simulink model "hw1"  (R2022a)
settings: Solver=VariableStepAuto  StartTime=0.0  StopTime=40  RelTol=1e-3
settings Model: Creator=谢嵩  LastModifiedBy=谢嵩

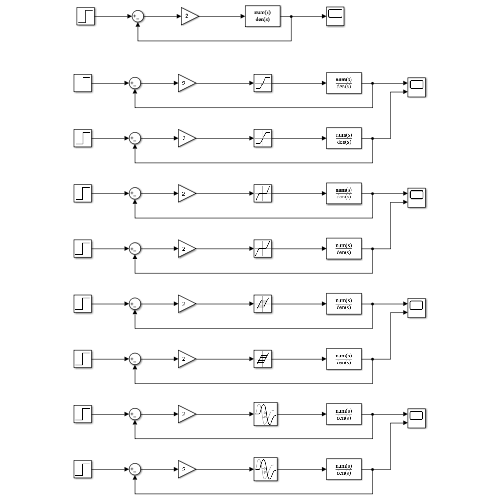
[thumbnail: Simulink's stored preview of the top-level diagram]
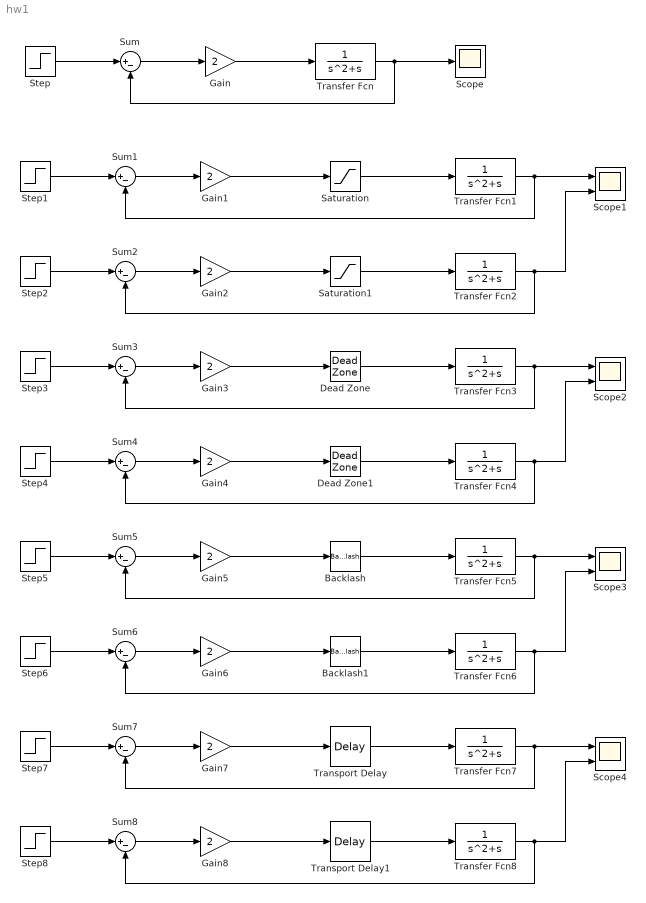
== system hw1 ==
  Backlash : Backlash
  Backlash1 : Backlash  BacklashWidth=0.4
  Dead Zone : DeadZone
  Dead Zone1 : DeadZone  LowerValue=-0.2  UpperValue=0.2
  Gain{,1..8} (9 alike) : Gain  Gain=2
  Saturation : Saturate
  Saturation1 : Saturate  UpperLimit=0.2  LowerLimit=-0.2
  Scope : Scope
  Scope{1..4} (4 alike) : Scope  NumInputPorts=2
  Step{,1..8} (9 alike) : Step  SampleTime=0
  Sum{,1..8} (9 alike) : Sum  Inputs=|+-
  Transfer Fcn{,1..8} (9 alike) : TransferFcn  Denominator=[1 1 0]
  Transport Delay : TransportDelay  DelayTime=0.5
  Transport Delay1 : TransportDelay  DelayTime=0.2
  wires:
  Step/1 -> Sum/1
  Sum/1 -> Gain/1
  Gain/1 -> Transfer Fcn/1
  Transfer Fcn/1 -> Sum/2, Scope/1
  Transfer Fcn1/1 -> Sum1/2, Scope1/1
  Step1/1 -> Sum1/1
  Sum1/1 -> Gain1/1
  Gain1/1 -> Saturation/1
  Saturation/1 -> Transfer Fcn1/1
  Transfer Fcn2/1 -> Scope1/2, Sum2/2
  Sum2/1 -> Gain2/1
  Saturation1/1 -> Transfer Fcn2/1
  Step2/1 -> Sum2/1
  Gain2/1 -> Saturation1/1
  Dead Zone/1 -> Transfer Fcn3/1
  Sum3/1 -> Gain3/1
  Transfer Fcn3/1 -> Sum3/2, Scope2/1
  Step3/1 -> Sum3/1
  Dead Zone1/1 -> Transfer Fcn4/1
  Transfer Fcn4/1 -> Scope2/2, Sum4/2
  Gain4/1 -> Dead Zone1/1
  Sum4/1 -> Gain4/1
  Step4/1 -> Sum4/1
  Gain3/1 -> Dead Zone/1
  Gain5/1 -> Backlash/1
  Backlash/1 -> Transfer Fcn5/1
  Backlash1/1 -> Transfer Fcn6/1
  Sum6/1 -> Gain6/1
  Step6/1 -> Sum6/1
  Gain6/1 -> Backlash1/1
  Step5/1 -> Sum5/1
  Transfer Fcn5/1 -> Sum5/2, Scope3/1
  Transfer Fcn6/1 -> Scope3/2, Sum6/2
  Sum5/1 -> Gain5/1
  Transport Delay/1 -> Transfer Fcn7/1
  Transfer Fcn7/1 -> Sum7/2, Scope4/1
  Step7/1 -> Sum7/1
  Transfer Fcn8/1 -> Scope4/2, Sum8/2
  Sum7/1 -> Gain7/1
  Sum8/1 -> Gain8/1
  Step8/1 -> Sum8/1
  Transport Delay1/1 -> Transfer Fcn8/1
  Gain7/1 -> Transport Delay/1
  Gain8/1 -> Transport Delay1/1
